simulink model "PMSM_FOC_DbComp_2017a"  (R2023b)
settings: Solver=ode23  StartTime=0.0  StopTime=0.1  FixedStep=1e-7  MaxStep=5e-7  RelTol=1e-3
libraries: slpidlib x4, spsDCVoltageSourceLib x2, spsUniversalBridgeLib x2, spsPermanentMagnetSynchronousMachineLib x2, simulink x2, sps_lib x1
(part 2 of 2)

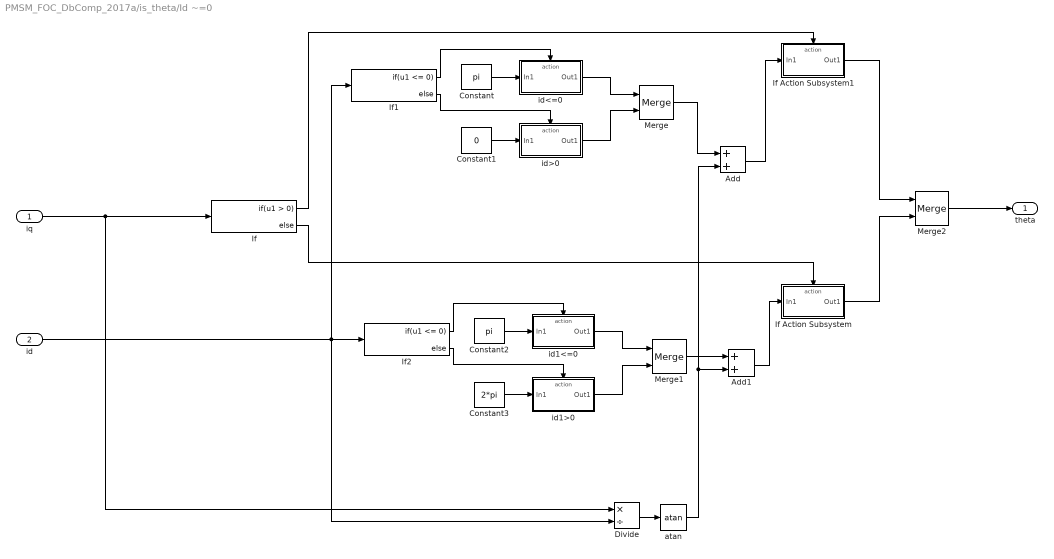
== system PMSM_FOC_DbComp_2017a/is_theta/Id ~=0 ==
  iq : Inport
  id : Inport  Port=2
  Add : Sum
  Add1 : Sum
  Constant : Constant  Value=pi
  Constant1 : Constant  Value=0
  Constant2 : Constant  Value=pi
  Constant3 : Constant  Value=2*pi
  Divide : Product  Inputs=*/
  If : If
  If Action Subsystem : Subsystem  TreatAsAtomicUnit=on
  If Action Subsystem1 : Subsystem  TreatAsAtomicUnit=on
  If1 : If  IfExpression=u1 <= 0
  If2 : If  IfExpression=u1 <= 0
  Merge : Merge
  Merge1 : Merge
  Merge2 : Merge
  atan : Trigonometry  Operator=atan
  id1<=0 : Subsystem  TreatAsAtomicUnit=on
  id1>0 : Subsystem  TreatAsAtomicUnit=on
  id<=0 : Subsystem  TreatAsAtomicUnit=on
  id>0 : Subsystem  TreatAsAtomicUnit=on
  theta : Outport
  wires:
  iq/1 -> If/1, Divide/1
  id/1 -> If1/1, Divide/2, If2/1
  If/1 -> If Action Subsystem1/Action
  If/2 -> If Action Subsystem/Action
  If1/1 -> id<=0/Action
  If1/2 -> id>0/Action
  id<=0/1(Out1) -> Merge/1
  id>0/1(Out1) -> Merge/2
  Constant/1 -> id<=0/1(In1)
  Constant1/1 -> id>0/1(In1)
  If2/1 -> id1<=0/Action
  If2/2 -> id1>0/Action
  id1<=0/1(Out1) -> Merge1/1
  id1>0/1(Out1) -> Merge1/2
  Constant2/1 -> id1<=0/1(In1)
  Constant3/1 -> id1>0/1(In1)
  If Action Subsystem1/1(Out1) -> Merge2/1
  If Action Subsystem/1(Out1) -> Merge2/2
  Divide/1 -> atan/1
  Merge2/1 -> theta/1
  Merge/1 -> Add/1
  atan/1 -> Add1/2, Add/2
  Add/1 -> If Action Subsystem1/1(In1)
  Merge1/1 -> Add1/1
  Add1/1 -> If Action Subsystem/1(In1)

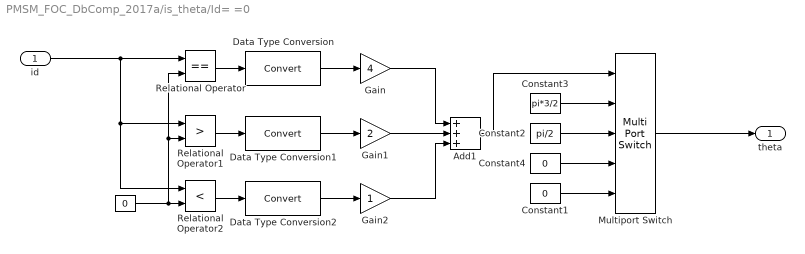
== system PMSM_FOC_DbComp_2017a/is_theta/Id= =0 ==
  id : Inport
  " " : Constant  Value=0
  Add1 : Sum  Inputs=+++
  Constant1 : Constant  Value=0
  Constant2 : Constant  Value=pi/2
  Constant3 : Constant  Value=pi*3/2
  Constant4 : Constant  Value=0
  Data Type Conversion : DataTypeConversion  SaturateOnIntegerOverflow=off  RndMeth=Floor
  Data Type Conversion1 : DataTypeConversion  SaturateOnIntegerOverflow=off  RndMeth=Floor
  Data Type Conversion2 : DataTypeConversion  SaturateOnIntegerOverflow=off  RndMeth=Floor
  Gain : Gain  Gain=4
  Gain1 : Gain  Gain=2
  Gain2 : Gain
  Multiport Switch : MultiPortSwitch  Inputs=4  SaturateOnIntegerOverflow=off  InputSameDT=off
  Relational Operator : RelationalOperator  Operator===  OutDataTypeStr=boolean  InputSameDT=off
  Relational Operator1 : RelationalOperator  Operator=>  OutDataTypeStr=boolean  InputSameDT=off
  Relational Operator2 : RelationalOperator  Operator=<  OutDataTypeStr=boolean  InputSameDT=off
  theta : Outport
  wires:
  Multiport Switch/1 -> theta/1
  Constant1/1 -> Multiport Switch/5
  Constant2/1 -> Multiport Switch/3
  Constant3/1 -> Multiport Switch/2
  id/1 -> Relational Operator2/1, Relational Operator1/1, Relational Operator/1
  " "/1 -> Relational Operator/2, Relational Operator1/2, Relational Operator2/2
  Relational Operator1/1 -> Data Type Conversion1/1
  Gain/1 -> Add1/1
  Gain2/1 -> Add1/3
  Add1/1 -> Multiport Switch/1
  Relational Operator/1 -> Data Type Conversion/1
  Relational Operator2/1 -> Data Type Conversion2/1
  Data Type Conversion/1 -> Gain/1
  Data Type Conversion1/1 -> Gain1/1
  Data Type Conversion2/1 -> Gain2/1
  Gain1/1 -> Add1/2
  Constant4/1 -> Multiport Switch/4

== system PMSM_FOC_DbComp_2017a/is_theta/If Action Subsystem ==
  In1 : Inport
  Action Port : ActionPort  ActionPortLabel=else
  Out1 : Outport
  wires:
  In1/1 -> Out1/1

== system PMSM_FOC_DbComp_2017a/is_theta/If Action Subsystem1 ==
  In1 : Inport
  Action Port : ActionPort  ActionPortLabel=if(u1 ~= 0)
  Out1 : Outport
  wires:
  In1/1 -> Out1/1

== system PMSM_FOC_DbComp_2017a/is_theta/Id ~=0/If Action Subsystem ==
  In1 : Inport
  Action Port : ActionPort  ActionPortLabel=else
  Out1 : Outport
  wires:
  In1/1 -> Out1/1

== system PMSM_FOC_DbComp_2017a/is_theta/Id ~=0/If Action Subsystem1 ==
  In1 : Inport
  Action Port : ActionPort  ActionPortLabel=if(u1 > 0)
  Out1 : Outport
  wires:
  In1/1 -> Out1/1

== system PMSM_FOC_DbComp_2017a/is_theta/Id ~=0/id1<=0 ==
  In1 : Inport
  Action Port : ActionPort  ActionPortLabel=if(u1 <= 0)
  Out1 : Outport
  wires:
  In1/1 -> Out1/1

== system PMSM_FOC_DbComp_2017a/is_theta/Id ~=0/id1>0 ==
  In1 : Inport
  Action Port : ActionPort  ActionPortLabel=else
  Out1 : Outport
  wires:
  In1/1 -> Out1/1

== system PMSM_FOC_DbComp_2017a/is_theta/Id ~=0/id<=0 ==
  In1 : Inport
  Action Port : ActionPort  ActionPortLabel=if(u1 <= 0)
  Out1 : Outport
  wires:
  In1/1 -> Out1/1

== system PMSM_FOC_DbComp_2017a/is_theta/Id ~=0/id>0 ==
  In1 : Inport
  Action Port : ActionPort  ActionPortLabel=else
  Out1 : Outport
  wires:
  In1/1 -> Out1/1
